simulink model "M_PSK"  (Simulink 7.7)
settings: Solver=ode45  StartTime=0.0  StopTime=10.0  RelTol=1e-3
values from neighbouring files (symbols this model uses):
  lengthOfSymbol = 64    [M_PSK_config.m]    (also in modulationen_config.m)
  sampleTime = 1    [M_PSK_config.m]    (also in modulationen_config.m)
undefined symbols (not defined in the file or in its folder): dfilt, fdesignblkfcn, gcbh, get
libraries: commsink2 x3, dsparch4 x2, commchan3 x1, commdigbbndpm3 x1, commutil2 x1, dspsigops x1
settings Model: Creator=mainster  LastModifiedBy=mainster

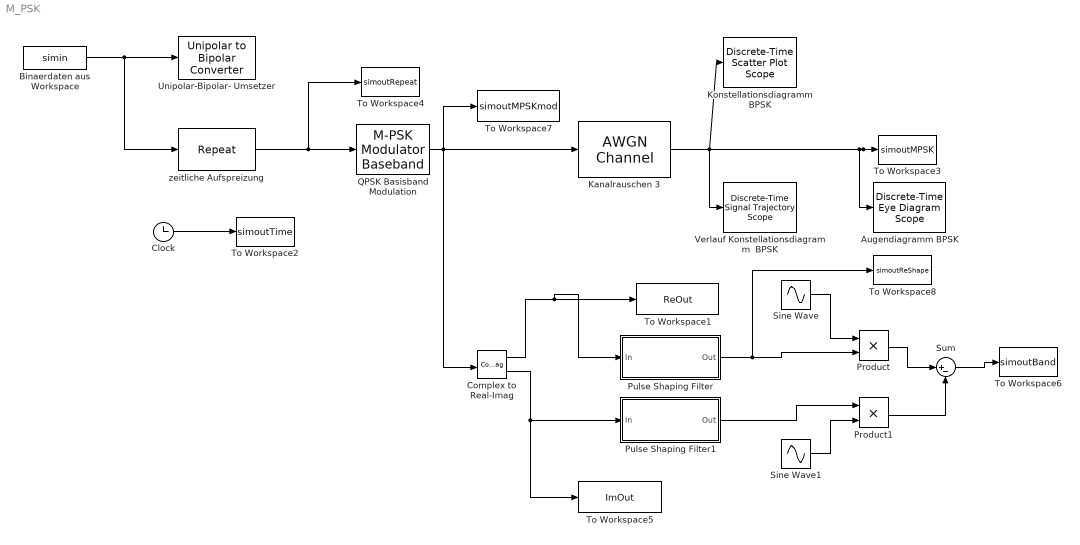
== system M_PSK ==
  Augendiagramm BPSK : commsink2/Discrete-Time Eye Diagram Scope  Tag=EyeDiagram  SystemSampleTime=-1  sampPerSymb=lengthOfSymbol  offsetEye=0  symbPerTrace=2  numTraces=40  numNewFrames=10  LineStyles=-  LineColors=b  dupPoints=on  fading=on  render=on  AxisGrid=on  yMin=-1.5  yMax=1.5  inphaseLabel=Amplitude Realteil  quadratureLabel=Amplitude Imaginaerteil  openScopeAtSimStart=on  dispDiagram=In-phase and Quadrature  FrameNumber=off  FigPos=get(0,'defaultfigureposition');  figTitle=Augendiagramm (2 Symbole)  block_type_=eye  numLinesMax=8
  Binaerdaten aus Workspace : FromWorkspace  VariableName=simin  SampleTime=sampleTime
  Clock : Clock
  Complex to Real-Imag : ComplexToRealImag
  Kanalrauschen 3 : commchan3/AWGN Channel  SystemSampleTime=-1  InputProcessing=Inherited (this choice will be removed - see release notes)  seed=67  noiseMode="Signal to noise ratio  (SNR)"  EbNodB=30  EsNodB=10  SNRdB=SNR  bitsPerSym=1  Ps=1  Tsym=1  variance=1
  Konstellationsdiagramm BPSK : commsink2/Discrete-Time Scatter Plot Scope  Tag=ScatterPlot  SystemSampleTime=-1  sampPerSymb=lengthOfSymbol  offsetEye=0  numTraces=150  numNewFrames=20  LineMarkers=.  LineColors=b  fading=on  render=on  AxisGrid=on  xMin=-1.3  xMax=1.315  yMin=-1.3  yMax=1.315  inphaseLabel=Amplitude Realteil  quadratureLabel=Amplitude Imaginaerteil  openScopeAtSimStart=on  FrameNumber=off  FigPos=[414 218 560 420]  figTitle=Konstellationsdiagramm  numLinesMax=8  block_type_=scatter
  Product : Product  RndMeth=Zero
  Product1 : Product  RndMeth=Zero
  Pulse Shaping Filter : Subsystem  DialogController=fdesignblkfcn  DialogControllerArgs=DataTag2  InitFcn=fdesignblkfcn(gcbh, {'InitFcn'});
      settings: CopyFcn=fdesignblkfcn(gcbh, {'CopyFcn'});
      mask Type: Pulse Shaping Filter
      mask Description: Design a Pulse Shaping Filter
      mask Help: helpview(mapfilelocation('dsp'), 'dsppulseshapingfilter');
      mask Display: disp('Pulse Shaping');
  Pulse Shaping Filter1 : Subsystem  DialogController=fdesignblkfcn  DialogControllerArgs=DataTag5  InitFcn=fdesignblkfcn(gcbh, {'InitFcn'});
      settings: CopyFcn=fdesignblkfcn(gcbh, {'CopyFcn'});
      mask Type: Pulse Shaping Filter
      mask Description: Design a Pulse Shaping Filter
      mask Help: helpview(mapfilelocation('dsp'), 'dsppulseshapingfilter');
      mask Display: disp('Pulse Shaping');
  QPSK Basisband Modulation : commdigbbndpm3/M-PSK Modulator Baseband  M=4  InType=Integer  Enc=Gray  Mapping=[0:2]  Ph=phaseOffset  outDtype=double  outWordLen=16  outUDDataType=sfix(16)  outFracLenMode=Best precision  outFracLen=15
  Sine Wave : Sin  Frequency=100  Phase=-pi/2  SampleTime=0
  Sine Wave1 : Sin  Frequency=00  SampleTime=0
  Sum : Sum  Inputs=|+-
  To Workspace1 : ToWorkspace  VariableName=ReOut  SampleTime=-1  SaveFormat=Structure
  To Workspace2 : ToWorkspace  VariableName=simoutTime  SampleTime=-1  SaveFormat=Structure
  To Workspace3 : ToWorkspace  VariableName=simoutMPSK  SampleTime=-1  SaveFormat=Structure
  To Workspace4 : ToWorkspace  VariableName=simoutRepeat  SampleTime=-1  SaveFormat=Structure
  To Workspace5 : ToWorkspace  VariableName=ImOut  SampleTime=-1  SaveFormat=Structure
  To Workspace6 : ToWorkspace  VariableName=simoutBand  SampleTime=-1  SaveFormat=Structure
  To Workspace7 : ToWorkspace  VariableName=simoutMPSKmod  SampleTime=-1  SaveFormat=Structure
  To Workspace8 : ToWorkspace  VariableName=simoutReShape  SampleTime=-1  SaveFormat=Structure
  Unipolar-Bipolar- Umsetzer : commutil2/Unipolar to Bipolar Converter  SystemSampleTime=-1  M=2  polarity=Positive  dataType=Inherit via internal rule
  Verlauf Konstellationsdiagramm  BPSK : commsink2/Discrete-Time Signal Trajectory Scope  Tag=SignalTrajectory  SystemSampleTime=-1  sampPerSymb=lengthOfSymbol  offsetEye=0  numTraces=40  numNewFrames=10  LineStyles=-  LineColors=b  fading=on  render=on  AxisGrid=on  xMin=-1.05  xMax=1.05  yMin=-1.05  yMax=1.05  inphaseLabel=Amplitude Realteil  quadratureLabel=Amplitude Imaginaerteil  openScopeAtSimStart=on  FrameNumber=off  FigPos=get(0,'defaultfigureposition');  figTitle=Verlauf Konstellationsdiagramm  numLinesMax=8  block_type_=xy
  zeitliche Aufspreizung : dspsigops/Repeat  N=lengthOfSymbol  InputProcessing=Inherited (this choice will be removed - see release notes)  RateOptions=Allow multirate processing  ic=0  mode=Unused parameter value
  wires:
  Binaerdaten aus Workspace/1 -> Unipolar-Bipolar- Umsetzer/1, zeitliche Aufspreizung/1
  Clock/1 -> To Workspace2/1
  QPSK Basisband Modulation/1 -> Kanalrauschen 3/1, To Workspace7/1, Complex to Real-Imag/1
  Kanalrauschen 3/1 -> To Workspace3/1, Augendiagramm BPSK/1, Konstellationsdiagramm BPSK/1, Verlauf Konstellationsdiagramm  BPSK/1
  zeitliche Aufspreizung/1 -> QPSK Basisband Modulation/1, To Workspace4/1
  Complex to Real-Imag/1 -> To Workspace1/1, Pulse Shaping Filter/1(In)
  Complex to Real-Imag/2 -> To Workspace5/1, Pulse Shaping Filter1/1(In)
  Pulse Shaping Filter1/1(Out) -> Product1/1
  Pulse Shaping Filter/1(Out) -> Product/2, To Workspace8/1
  Sine Wave/1 -> Product/1
  Sine Wave1/1 -> Product1/2
  Product/1 -> Sum/1
  Product1/1 -> Sum/2
  Sum/1 -> To Workspace6/1

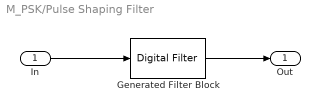
== system M_PSK/Pulse Shaping Filter ==
  In : Inport
  Generated Filter Block : dsparch4/Digital Filter  Tag=BlockMethodSubSystem  TypePopup=FIR (all zeros)  IIRFiltStruct=Direct form II transposed  AllPoleFiltStruct=Direct form  FIRFiltStruct=Direct form  CoeffSource=Specify via dialog  NumCoeffs=[-1.90327561986829e-05 -1.55646542059928e-05 -1.19994648576602e-05 -8.35663458843645e-06 -4.65613689415661e-06 -9.1836266130336e-07 2.83599245861524e-06 6.58604301165962e-06 1.03108304060328e-05 1.39894406303172e-05 1.76011223673135e-05 2.11254048393332e-05 2.45422147183864e-05 2.78319914360779e-05 3.09758002330938e-05 3.39554422970383e-05 3.67535613499344e-05 3.93537460629507e-05 4.17406276957613e-05 4.38999723813093e-05 4.58187675035094e-05 4.74853016454643e-05 4.88892376189325e-05 5.00216781219151e-05 5.08752236101153e-05 5.14440220095015e-05 5.17238099410163e-05 5.17119451744239e-05 5.1407430076101e-05 5.08109258650191e-05 4.99247575419481e-05 4.87529094087816e-05 4.73010111475254e-05 4.55763144816473e-05 4.35876604958286e-05 4.13454377434114e-05 3.88615313236947e-05 3.61492631633789e-05 3.32233237876297e-05 3.00996959160975e-05 2.67955702675264e-05 2.33292540030234e-05 1.97200722823462e-05 1.59882634495027e-05 1.21548684031814e-05 8.24161474393995e-06 4.27079632332336e-06 2.65148850054405e-07 -3.75227776511228e-06 -7.7582496215136e-06 -1.17294808743577e-05 -1.56427668758578e-05 -1.94751176624862e-05 -2.32038910323528e-05 -2.68069244541667e-05 -3.02626650509472e-05 -3.35502969076589e-05 -3.66498649622042e-05 -3.95423947537374e-05 -4.22100073209643e-05 -4.46360285659109e-05 -4.6805092425492e-05 -4.87032372239173e-05 -5.0317994613452e-05 -5.16384705490708e-05 -5.26554177839709e-05 -5.33612994174978e-05 -5.37503430745632e-05 -5.38185853458658e-05 -5.35639061708765e-05 -5.29860529003576e-05 -5.20866538318453e-05 -5.08692210697386e-05 -4.93391426210789e-05 -4.75036636984674e-05 -4.53718572624811e-05 -4.29545838971262e-05 -4.02644411729169e-05 -3.73157027127716e-05 -3.41242472357467e-05 -3.07074779122798e-05 -2.70842324218491e-05 -2.32746841593236e-05 -1.93002350895729e-05 -1.51834008007142e-05 -1.09476883544632e-05 -6.61746757710333e-06 -2.21783647630999e-06 2.22551849274799e-06 6.68646655426146e-06 1.11385803434738e-05 1.55552864289938e-05 1.99100177898147e-05 2.41763673939414e-05 2.83282420131018e-05 3.23400154003e-05 3.61866799541831e-05 3.98439959962762e-05 4.32886377941814e-05 4.64983354758225e-05 4.94520119966796e-05 5.21299143436905e-05 5.45137381859697e-05 5.65867452136206e-05 5.83338724415442e-05 5.97418327951013e-05 6.07992063385984e-05 6.14965215555875e-05 6.18263261416944e-05 6.17832468258223e-05 6.13640377938543e-05 6.05676173500927e-05 5.93950925152969e-05 5.78497713259778e-05 5.59371626672389e-05 5.36649635405258e-05 5.10430337378121e-05 4.80833579646084e-05 4.47999955253393e-05 4.12090177557108e-05 3.73284334572609e-05 3.3178102658983e-05 2.87796390993171e-05 2.41563018885138e-05 1.93328768760588e-05 1.43355483100259e-05 9.19176143467368e-06 3.93007672879711e-06 -1.41998345988149e-06 -6.82809508010212e-06 -1.22632984932836e-05 -1.76941696512031e-05 -2.30889954101176e-05 -2.8415952025465e-05 -3.36432858456334e-05 -3.87394952028857e-05 -4.36735124845964e-05 -4.84148853586291e-05 -5.29339561229856e-05 -5.72020381519474e-05 -6.11915884187582e-05 -6.48763750885233e-05 -6.82316391943724e-05 -7.1234249434957e-05 -7.38628491620156e-05 -7.60979946628102e-05 -7.7922283883652e-05 -7.93204747872332e-05 -8.02795925878899e-05 -8.07890251649742e-05 -8.0840606014931e-05 -8.04286841671702e-05 -7.95501805570542e-05 -7.82046304209463e-05 -7.63942113529097e-05 -7.41237567399144e-05 -7.1400754371902e-05 -6.82353301043396e-05 -6.46402165335277e-05 -6.06307067284722e-05 -5.6224593147124e-05 -5.14420919487498e-05 -4.63057529977094e-05 -4.08403559364182e-05 -3.50727927864284e-05 -2.90319376157652e-05 -2.27485038875584e-05 -1.62548901791238e-05 -9.58501503152397e-06 -2.77414175689823e-06 4.14130590596972e-06 1.11239363385925e-05 1.81355897889973e-05 2.51375442651718e-05 3.20907264802518e-05 3.89559267163567e-05 4.56940164422448e-05 5.22661674945539e-05 5.86340716133246e-05 6.47601591100052e-05 7.06078154403954e-05 7.61415944559119e-05 8.13274271144439e-05 8.61328244466814e-05 9.05270735953197e-05 9.44814257727677e-05 ...(+23512 chars)]  DenCoeffs=[1 0.1]  BiQuadCoeffs=[1 0.3 0.4 1 0.1 0.2]  LatticeCoeffs=[0.2 0.4]  denIgnore=on  FiltPerSampPopup=One filter per frame  IC=0  ICnum=0  ICden=0  roundingMode=Floor  overflowMode=off  ScaleValues=1  scaleValueFracLength=14  stageInFracLength=15  stageOutFracLength=15  FilterSource=Specify via dialog  dfiltObjectName=dfilt.dffir([1 2 1])  InputProcessing=Columns as channels (frame based)
  Out : Outport
  wires:
  In/1 -> Generated Filter Block/1
  Generated Filter Block/1 -> Out/1

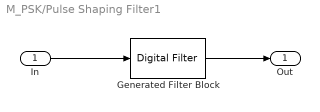
== system M_PSK/Pulse Shaping Filter1 ==
  In : Inport
  Generated Filter Block : dsparch4/Digital Filter  Tag=BlockMethodSubSystem  TypePopup=FIR (all zeros)  IIRFiltStruct=Direct form II transposed  AllPoleFiltStruct=Direct form  FIRFiltStruct=Direct form  CoeffSource=Specify via dialog  NumCoeffs=[0.000556485815006627 0.00047310526441413 0.000211846817044442 -0.000154939970550363 -0.000511543361452901 -0.000734999783432546 -0.000737042578549377 -0.000498021416956038 -8.0381284389844e-05 0.000384913318275134 0.000737042578549378 0.000838377586982178 0.000625219663997989 0.000138588892479704 -0.000477693803139429 -0.00101469588358633 -0.0012631344689833 -0.00108635852051072 -0.000477693803139427 0.000419352168569643 0.00133975642285284 0.0019714069018707 0.00205650341846994 0.00148961892805067 0.000378940340694988 -0.000955547365643391 -0.00205650341846994 -0.00246382372206811 -0.00187565899199397 -0.000288335862807293 0.00193352253651673 0.00409196438091809 0.00530516476972985 0.00474842520200766 0.00193352253651673 -0.0030460800545258 -0.00937829495996986 -0.0155594464116502 -0.0196053325894134 -0.0194213065481005 -0.0132629119243246 -0.000188227193533446 0.0196053325894134 0.0446496234889096 0.0723290587040688 0.0992526582797615 0.121811919800554 0.136816456118228 0.142077471545948 0.136816456118228 0.121811919800554 0.0992526582797615 0.0723290587040688 0.0446496234889096 0.0196053325894134 -0.000188227193533446 -0.0132629119243246 -0.0194213065481005 -0.0196053325894134 -0.0155594464116502 -0.00937829495996986 -0.0030460800545258 0.00193352253651673 0.00474842520200766 0.00530516476972985 0.00409196438091809 0.00193352253651673 -0.000288335862807293 -0.00187565899199397 -0.00246382372206811 -0.00205650341846994 -0.000955547365643391 0.000378940340694988 0.00148961892805067 0.00205650341846994 0.0019714069018707 0.00133975642285284 0.000419352168569643 -0.000477693803139427 -0.00108635852051072 -0.0012631344689833 -0.00101469588358633 -0.000477693803139429 0.000138588892479704 0.000625219663997989 0.000838377586982178 0.000737042578549378 0.000384913318275134 -8.0381284389844e-05 -0.000498021416956038 -0.000737042578549377 -0.000734999783432546 -0.000511543361452901 -0.000154939970550363 0.000211846817044442 0.00047310526441413 0.000556485815006627]  DenCoeffs=[1 0.1]  BiQuadCoeffs=[1 0.3 0.4 1 0.1 0.2]  LatticeCoeffs=[0.2 0.4]  denIgnore=on  FiltPerSampPopup=One filter per frame  IC=0  ICnum=0  ICden=0  roundingMode=Floor  overflowMode=off  ScaleValues=1  scaleValueFracLength=14  stageInFracLength=15  stageOutFracLength=15  FilterSource=Specify via dialog  dfiltObjectName=dfilt.dffir([1 2 1])  InputProcessing=Columns as channels (frame based)
  Out : Outport
  wires:
  In/1 -> Generated Filter Block/1
  Generated Filter Block/1 -> Out/1
